simulink model "DescreteModel"  (R2020b)
settings: Solver=FixedStepAuto  StartTime=0.0  StopTime=3  FixedStep=0.0001  RelTol=1e-3
values from neighbouring files (symbols this model uses):
  B = 3.4    [NonLinearModelParameters.m]
  J_eq = J_1 + n_1^2 *(J_2 + M_3*r_3^2)    (= 2.88733377778e-05)    [NonLinearModelParameters.m]
  K_tau = 42e-3    (= 0.042)    [NonLinearModelParameters.m]
  n_1 = 1/3    (= 0.333333333333)    [NonLinearModelParameters.m]
  r_3 = 0.0127    [NonLinearModelParameters.m]
  T_sample = 0.001    [NonLinearModelParameters.m]
undefined symbols (not defined in the file or in its folder): CoulombAndViscousFriction
settings Model: Creator=jonas  LastModifiedBy=jonas

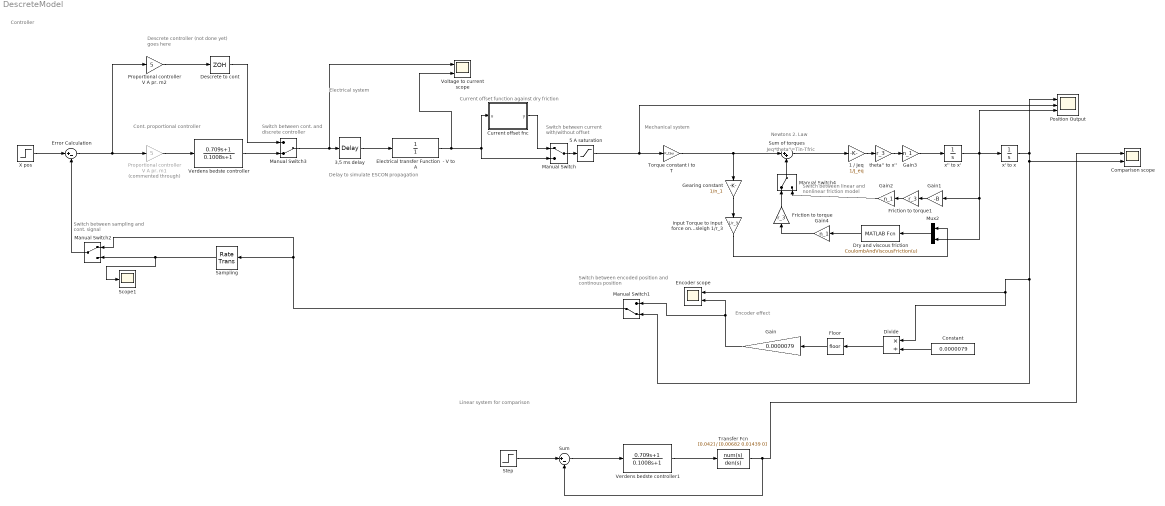
== system DescreteModel ==
  note: Linear system for comparison
  note: Switch between linear
      | and nonlinear friction model
  note: Delay to simulate ESCON propagation
  note: Switch between
      | current with/without offset
  note: Switch between sampling
      | and cont. signal
  note: Controller
  note: Electrical system
  note: Switch between cont.
      | and discrete controller
  note: Current offset function against dry friction
  note: Cont. proportional
      | controller
  note: Switch between encoded position and
      | continous position
  note: Newtons 2. Law
  note: Mechanical system
  note: Encoder effect
  note: Jeq*theta''=Tin-Tfric
  note: Descrete controller (not done yet) goes here
  1 / Jeq : Gain  Gain=1/J_eq
  3,5 ms delay : TransportDelay  DelayTime=0.0035
  5 A saturation : Saturate  UpperLimit=5  LowerLimit=-5
  Comparison scope : Scope  NumInputPorts=2
  Constant : Constant  Value=0.0000079
  Current offset fnc : MATLAB Function  TreatAsAtomicUnit=on
  Descrete to cont : ZeroOrderHold  SampleTime=T_sample
  Divide : Product  Inputs=*/
  Dry and viscous friction : MATLABFcn  MATLABFcn=CoulombAndViscousFriction(u)  OutputDimensions=1
  Electrical transfer Function  - V to A : TransferFcn  Denominator=[1]
  Encoder scope : Scope  NumInputPorts=2
  Error Calculation : Sum  Inputs=|+-
  Floor : Rounding
  Friction to torque : Gain  Gain=r_3
  Friction to torque1 : Gain  Gain=r_3
  Gain : Gain  Gain=0.0000079
  Gain1 : Gain  Gain=-B
  Gain2 : Gain  Gain=n_1
  Gain3 : Gain  Gain=n_1
  Gain4 : Gain  Gain=n_1
  Gearing constant : Gain  Gain=1/n_1
  Input Torque to input force on sleigh 1/r_3 : Gain  Gain=1/r_3
  Manual Switch : ManualSwitch
  Manual Switch1 : ManualSwitch  CurrentSetting=0
  Manual Switch2 : ManualSwitch
  Manual Switch3 : ManualSwitch  CurrentSetting=0
  Manual Switch4 : ManualSwitch
  Mux2 : Mux  Inputs=2
  Position Output : Scope  NumInputPorts=3
  Proportional controller V A pr. m1 : Gain  Commented=through  Gain=5
  Proportional controller V A pr. m2 : Gain  Gain=5
  "Sampling " : RateTransition  OutPortSampleTime=T_sample
  Scope1 : Scope
  Step : Step  Time=0  SampleTime=0
  Sum : Sum  Inputs=|+-
  Sum of torques : Sum  Inputs=|++
  "Torque constant I to T " : Gain  Gain=K_tau
  Transfer Fcn : TransferFcn  Numerator=[0.042]  Denominator=[0.00682 0.01439 0]
  Verdens bedste controller : TransferFcn  Numerator=[0.709 1]  Denominator=[0.1008 1]
  Verdens bedste controller1 : TransferFcn  Numerator=[0.709 1]  Denominator=[0.1008 1]
  Voltage to current scope : Scope  NumInputPorts=2
  X pos : Step  Time=0  SampleTime=0
  theta'' to x'' : Gain  Gain=r_3
  x' to x : Integrator
  x'' to x' : Integrator
  wires:
  Sum of torques/1 -> 1 / Jeq/1
  theta'' to x''/1 -> Gain3/1
  X pos/1 -> Error Calculation/1
  x'' to x'/1 -> Position Output/3, Gain1/1, Mux2/2, x' to x/1
  Manual Switch/1 -> 5 A saturation/1
  Input Torque to input force on sleigh 1/r_3/1 -> Mux2/1
  Mux2/1 -> Dry and viscous friction/1
  Current offset fnc/1(y) -> Manual Switch/1
  5 A saturation/1 -> Position Output/2, "Torque constant I to T "/1
  x' to x/1 -> Divide/1, Encoder scope/1, Manual Switch1/2, Comparison scope/2, Position Output/1
  Gain/1 -> Encoder scope/2, Manual Switch1/1
  Floor/1 -> Gain/1
  Constant/1 -> Divide/2
  Manual Switch3/1 -> 3,5 ms delay/1, Voltage to current scope/1
  Divide/1 -> Floor/1
  Manual Switch2/1 -> Error Calculation/2
  Manual Switch1/1 -> "Sampling "/1, Manual Switch2/1
  "Sampling "/1 -> Scope1/1, Manual Switch2/2
  Descrete to cont/1 -> Manual Switch3/1
  Proportional controller V A pr. m1/1 -> Verdens bedste controller/1
  Error Calculation/1 -> Proportional controller V A pr. m1/1, Proportional controller V A pr. m2/1
  Dry and viscous friction/1 -> Gain4/1
  Electrical transfer Function  - V to A/1 -> Current offset fnc/1(u), Manual Switch/2, Voltage to current scope/2
  3,5 ms delay/1 -> Electrical transfer Function  - V to A/1
  1 / Jeq/1 -> theta'' to x''/1
  Proportional controller V A pr. m2/1 -> Descrete to cont/1
  Verdens bedste controller/1 -> Manual Switch3/2
  Manual Switch4/1 -> Sum of torques/2
  Friction to torque/1 -> Manual Switch4/1
  Gain1/1 -> Friction to torque1/1
  Friction to torque1/1 -> Gain2/1
  Step/1 -> Sum/1
  Sum/1 -> Verdens bedste controller1/1
  Verdens bedste controller1/1 -> Transfer Fcn/1
  Transfer Fcn/1 -> Comparison scope/1, Sum/2
  "Torque constant I to T "/1 -> Sum of torques/1, Gearing constant/1
  Gearing constant/1 -> Input Torque to input force on sleigh 1/r_3/1
  Gain2/1 -> Manual Switch4/2
  Gain3/1 -> x'' to x'/1
  Gain4/1 -> Friction to torque/1

== matlab function DescreteModel/Current offset fnc ==
  data: u input; y output
function y = fcn(u)
if abs(u) < 1e-2;
    y=0;
else
y = u+(sign(u)*0.745);
end
